simulink model "Quad_IGE_Landing"  (R2023b)
settings: Solver=ode4  StartTime=0.0  StopTime=20  FixedStep=0.01  RelTol=1e-3
InitFcn:
  | m = 0.063;
  | g = 9.81;
  | R = 0.033;
  | h_r = 0.013;
  | b = 0.2;
libraries: simulink x2
settings Model: Creator=reza  LastModifiedBy=Ali
settings OptimizationCC: ReuseModelBlockBuffer=off

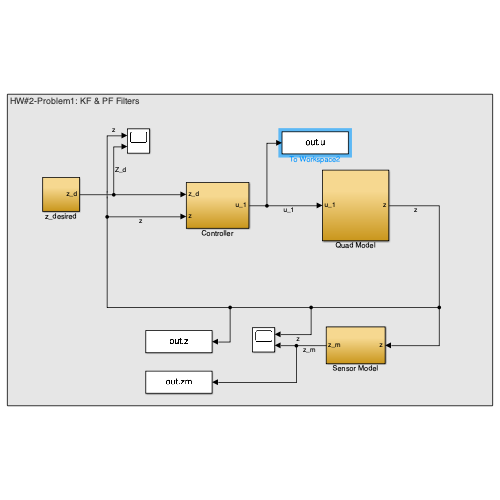
[thumbnail: Simulink's stored preview of the top-level diagram]
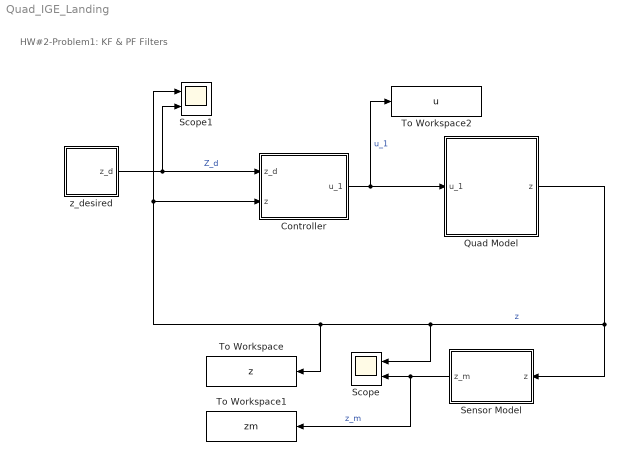
== system Quad_IGE_Landing ==
  note: HW#2-Problem1: KF & PF Filters
  Controller : Subsystem
  Quad Model : Subsystem
  Scope : Scope  NumInputPorts=2
  Scope1 : Scope  NumInputPorts=2
  Sensor Model : Subsystem
  To Workspace : ToWorkspace  VariableName=z  SaveFormat=Timeseries  SampleTime=-1
  To Workspace1 : ToWorkspace  VariableName=zm  SaveFormat=Timeseries  SampleTime=-1
  To Workspace2 : ToWorkspace  VariableName=u  SaveFormat=Timeseries  SampleTime=-1
  z_desired : Subsystem
  wires:
  Quad Model/1(z) -> Scope/1, To Workspace/1, Scope1/1, Controller/2(z), Sensor Model/1(z)  "z"
  z_desired/1(z_d) -> Scope1/2, Controller/1(z_d)  "Z_d"
  Sensor Model/1(z_m) -> To Workspace1/1, Scope/2  "z_m"
  Controller/1(u_1) -> To Workspace2/1, Quad Model/1(u_1)  "u_1"

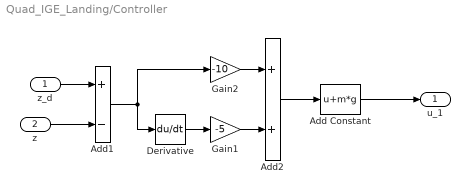
== system Quad_IGE_Landing/Controller ==
  z_d : Inport
  z : Inport  Port=2
  Add Constant : Bias  Bias=m*g  SaturateOnIntegerOverflow=off
  Add1 : Sum  Inputs=+-
  Add2 : Sum
  Derivative : Derivative
  Gain1 : Gain  Gain=-5
  Gain2 : Gain  Gain=-10
  u_1 : Outport
  wires:
  Gain1/1 -> Add2/2
  Add2/1 -> Add Constant/1
  z_d/1 -> Add1/1
  Add1/1 -> Gain2/1, Derivative/1
  Gain2/1 -> Add2/1
  Derivative/1 -> Gain1/1
  Add Constant/1 -> u_1/1
  z/1 -> Add1/2

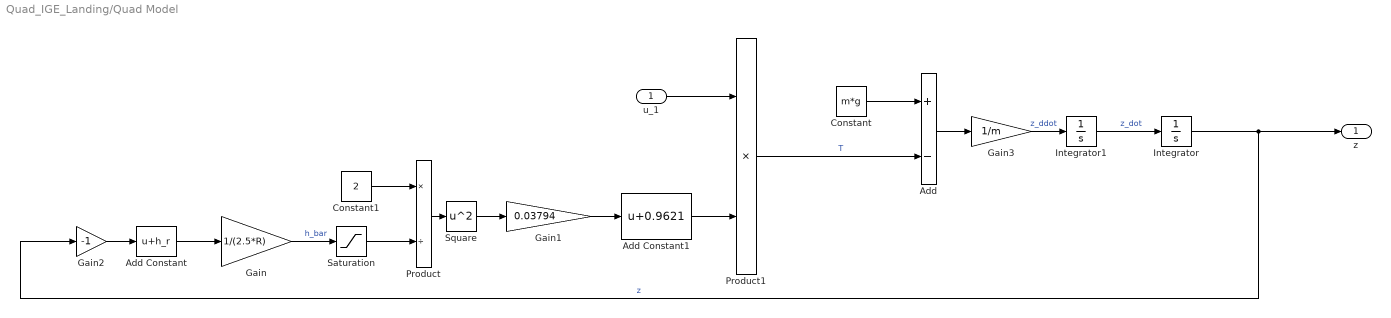
== system Quad_IGE_Landing/Quad Model ==
  u_1 : Inport
  Add : Sum  Inputs=+-
  Add Constant : Bias  Bias=h_r  SaturateOnIntegerOverflow=off
  Add Constant1 : Bias  Bias=0.9621  SaturateOnIntegerOverflow=off
  Constant : Constant  Value=m*g
  Constant1 : Constant  Value=2
  Gain : Gain  Gain=1/(2.5*R)
  Gain1 : Gain  Gain=0.03794
  Gain2 : Gain  Gain=-1
  Gain3 : Gain  Gain=1/m
  Integrator : Integrator  InitialCondition=-2
  Integrator1 : Integrator
  Product : Product  Inputs=*/
  Product1 : Product
  Saturation : Saturate  UpperLimit=2  LowerLimit=0
  Square : Math  Operator=square
  z : Outport
  wires:
  Saturation/1 -> Product/2
  Integrator1/1 -> Integrator/1  "z_dot"
  Gain/1 -> Saturation/1  "h_bar"
  Add/1 -> Gain3/1
  Add Constant/1 -> Gain/1
  Integrator/1 -> Gain2/1, z/1  "z"
  Gain1/1 -> Add Constant1/1
  Product/1 -> Square/1
  Square/1 -> Gain1/1
  Add Constant1/1 -> Product1/2
  Constant/1 -> Add/1
  Constant1/1 -> Product/1
  Product1/1 -> Add/2  "T"
  u_1/1 -> Product1/1
  Gain2/1 -> Add Constant/1
  Gain3/1 -> Integrator1/1  "z_ddot"

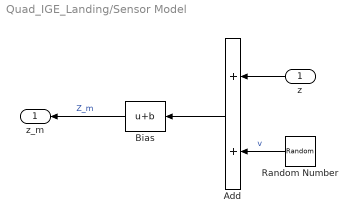
== system Quad_IGE_Landing/Sensor Model ==
  z : Inport
  Add : Sum
  Bias : Bias  Bias=b  SaturateOnIntegerOverflow=off
  Random Number : RandomNumber  Variance=0.1  SampleTime=0.01
  z_m : Outport
  wires:
  Random Number/1 -> Add/2  "v"
  Add/1 -> Bias/1
  z/1 -> Add/1
  Bias/1 -> z_m/1  "Z_m"

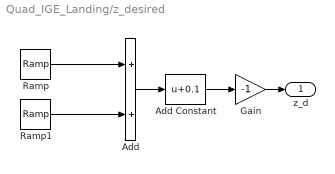
== system Quad_IGE_Landing/z_desired ==
  Add : Sum
  Add Constant : Bias  Bias=0.1  SaturateOnIntegerOverflow=off
  Gain : Gain  Gain=-1
  Ramp : simulink/Sources/Ramp  slope=-(2-0.1)/5  start=10  InitialOutput=2-0.1
  Ramp1 : simulink/Sources/Ramp  slope=(2-0.1)/5  start=15  InitialOutput=0
  z_d : Outport
  wires:
  Add Constant/1 -> Gain/1
  Ramp1/1 -> Add/2
  Ramp/1 -> Add/1
  Add/1 -> Add Constant/1
  Gain/1 -> z_d/1
